simulink model "lever"  (R2013a)
settings: Solver=ode45  StartTime=0.0  StopTime=10.0  RelTol=1e-3
settings Model: Creator=Ahmed  LastModifiedBy=Ahmed

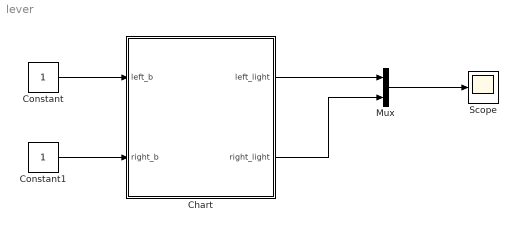
== system lever ==
  Chart : Stateflow chart  TreatAsAtomicUnit=on
  Constant : Constant
  Constant1 : Constant
  Mux : Mux  Inputs=2
  Scope : Scope
  wires:
  Constant/1 -> Chart/1(left_b)
  Constant1/1 -> Chart/2(right_b)
  Chart/1(left_light) -> Mux/1
  Chart/2(right_light) -> Mux/2
  Mux/1 -> Scope/1

== stateflow chart lever/Chart ==
  state OFF
    entry:
    left_light=0;
    right_light=0;
  state RIGHT
    state ON
      entry:
      right_light=1;
    state OFF
      entry:
      right_light=0;
    (default) -> RIGHT.ON
    RIGHT.OFF -> RIGHT.ON : after(0.5,sec)
    RIGHT.ON -> RIGHT.OFF : after(0.5,sec)
  state LEFT
    state ON
      entry:
      left_light=1;
    state OFF
      entry:
      left_light=0;
    (default) -> LEFT.ON
    LEFT.OFF -> LEFT.ON : after(0.5,sec)
    LEFT.ON -> LEFT.OFF : after(0.5,sec)
  (default) -> OFF
  LEFT -> OFF : [right_b==0&&left_b==0]
  RIGHT -> OFF : [right_b==0&&left_b==0]
  OFF -> LEFT [order 2] : [right_b==0&&left_b==1]
  OFF -> RIGHT [order 1] : [right_b==1&&left_b==0]
  data: left_b input; right_b input; left_light output double; right_light output double
